simulink model "robust_tracking_integral_REALTIME"  (R2020b)
settings: Solver=ode3  StartTime=0.0  StopTime=5  FixedStep=0.001  RelTol=1e-3
values from neighbouring files (symbols this model uses):
  ctrl =     [PID_params_LAB0.mat]
undefined symbols (not defined in the file or in its folder): degs2rpm, denH1, DiscIntNeverNeededParam, Ke, Ki, N_u, N_x, National_Instruments, numH1, PCI, rpm2rads, sens, step_size
libraries: sldrtlib x3, simulink x2
settings Model: ExtModeTrigDuration=10000  Creator=39345  LastModifiedBy=tortoranic
settings DataIOCC: ReturnWorkspaceOutputs=off
settings RTWCC: Description=Simulink Desktop Real-Time  SystemTargetFile=sldrt.tlc  TemplateMakefile=sldrt.tmf  RTWCompilerOptimization=on
settings CodeAppCC: MaxIdLength=95
settings SimulinkDesktopRealTimeCC: TargetPreCompLibLocation=C:\Program Files\MATLAB\R2020b\toolbox\sldrt\lib\win64

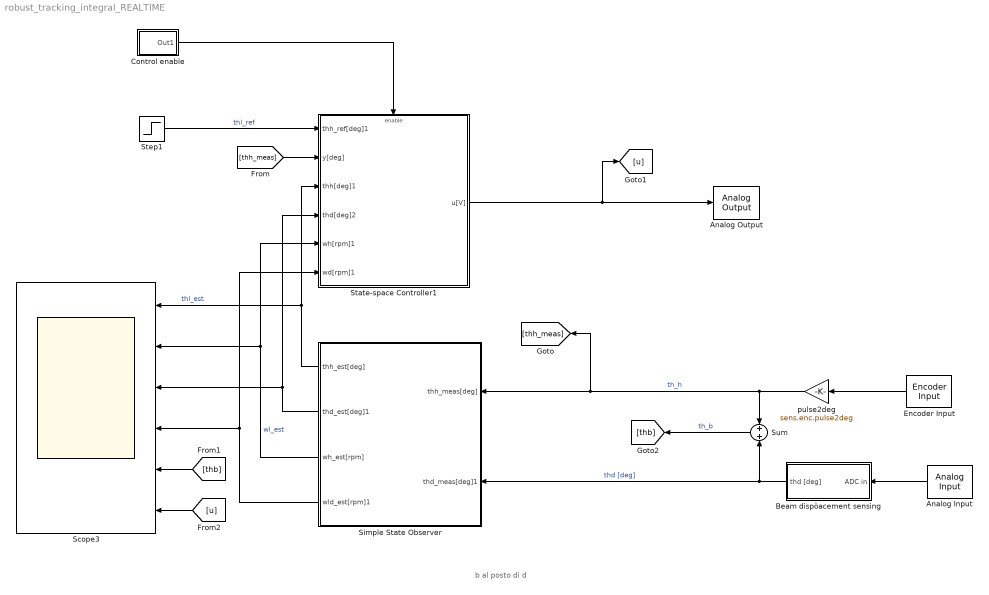
== system robust_tracking_integral_REALTIME ==
  note: b al posto di d
  Analog Input : sldrtlib/Analog Input  SampleTime=0.001  MaxMissedTicks=10  ShowMissedTicks=off  YieldWhenWaiting=off  DrvName=National_Instruments/PCI-6221  DrvAddress=4294967295  DrvOptions=[0 0 0 2 0]  Channels=[3 4]  RangeMode=1  VoltRange=2  DataType=1
      settings: AttributesFormatString=National Instruments\nPCI-6221 [auto]
  Analog Output : sldrtlib/Analog Output  SampleTime=0.001  MaxMissedTicks=10  ShowMissedTicks=off  YieldWhenWaiting=off  DrvName=National_Instruments/PCI-6221  DrvAddress=4294967295  DrvOptions=[0 0 0 2 0]  Channels=1  RangeMode=1  VoltRange=1  InitialValue=0  FinalValue=0
      settings: AttributesFormatString=National Instruments\nPCI-6221 [auto]
  Beam dispòacement sensing : Subsystem
  Control enable : Subsystem
  Encoder Input : sldrtlib/Encoder Input  SampleTime=0.001  MaxMissedTicks=10  ShowMissedTicks=off  YieldWhenWaiting=off  DrvName=National_Instruments/PCI-6221  DrvAddress=4294967295  DrvOptions=[0 0 0 2 0]  Channels=1  QuadMode=3  IndexPulse=1  InputFilter=Inf  DataType=1
      settings: AttributesFormatString=National Instruments\nPCI-6221 [auto]
  Scope3 : Scope  NumInputPorts=6
  Simple State Observer : Subsystem
  State-space Controller1 : Subsystem
  Step1 : Step  After=step_size  SampleTime=0.001
  Sum : Sum
  pulse2deg : Gain  Gain=sens.enc.pulse2deg
  wires:
  Simple State Observer/4(wld_est[rpm]1) -> Scope3/4, State-space Controller1/6(wd[rpm]1)
  Simple State Observer/1(thh_est[deg]) -> Scope3/1, State-space Controller1/3(thh[deg]1)  "thl_est"
  Simple State Observer/3(wh_est[rpm]) -> State-space Controller1/5(wh[rpm]1), Scope3/2  "wl_est"
  Simple State Observer/2(thd_est[deg]1) -> Scope3/3, State-space Controller1/4(thd[deg]2)
  Encoder Input/1 -> pulse2deg/1
  Sum/1 -> [thb]  "th_b"
  [thh_meas] -> State-space Controller1/2(y[deg])
  Step1/1 -> State-space Controller1/1(thh_ref[deg]1)  "thl_ref"
  State-space Controller1/1(u[V]) -> [u], Analog Output/1
  pulse2deg/1 -> Sum/1, [thh_meas], Simple State Observer/1(thh_meas[deg])  "th_h"
  Analog Input/1 -> Beam dispòacement sensing/1(ADC in)
  Beam dispòacement sensing/1(thd [deg]) -> Simple State Observer/2(thd_meas[deg]1), Sum/2  "thd [deg]"
  [thb] -> Scope3/5
  [u] -> Scope3/6
  Control enable/1(Out1) -> State-space Controller1/Enable

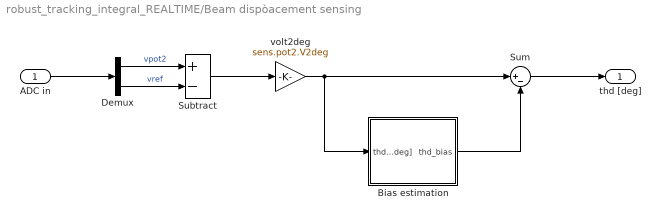
== system robust_tracking_integral_REALTIME/Beam dispòacement sensing ==
  ADC in : Inport
  Bias estimation : Subsystem
  Demux : Demux  Outputs=2
  Subtract : Sum  Inputs=+-
  Sum : Sum  Inputs=|+-
  volt2deg : Gain  Gain=sens.pot2.V2deg
  thd [deg] : Outport
  wires:
  Subtract/1 -> volt2deg/1
  Demux/1 -> Subtract/1  "vpot2"
  Demux/2 -> Subtract/2  "vref"
  ADC in/1 -> Demux/1
  volt2deg/1 -> Bias estimation/1(thd [deg]), Sum/1
  Bias estimation/1(thd_bias) -> Sum/2
  Sum/1 -> thd [deg]/1

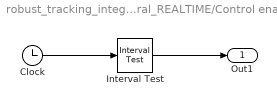
== system robust_tracking_integral_REALTIME/Control enable ==
  Clock : Clock
  Interval Test : simulink/Logic and Bit Operations/Interval Test  IntervalClosedRight=on  uplimit=60  IntervalClosedLeft=on  lowlimit=0.7  OutDataTypeStr=boolean
  Out1 : Outport
  wires:
  Clock/1 -> Interval Test/1
  Interval Test/1 -> Out1/1

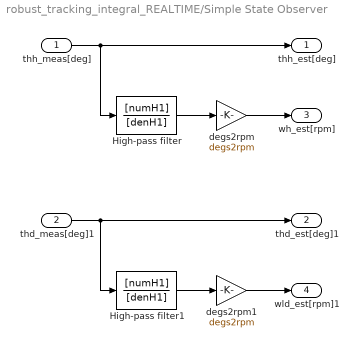
== system robust_tracking_integral_REALTIME/Simple State Observer ==
  thh_meas[deg] : Inport
  thd_meas[deg]1 : Inport  Port=2
  High-pass filter : TransferFcn  Numerator=[numH1]  Denominator=[denH1]
  High-pass filter1 : TransferFcn  Numerator=[numH1]  Denominator=[denH1]
  degs2rpm : Gain  Gain=degs2rpm
  degs2rpm1 : Gain  Gain=degs2rpm
  thh_est[deg] : Outport
  thd_est[deg]1 : Outport  Port=2
  wh_est[rpm] : Outport  Port=3
  wld_est[rpm]1 : Outport  Port=4
  wires:
  thh_meas[deg]/1 -> thh_est[deg]/1, High-pass filter/1
  High-pass filter/1 -> degs2rpm/1
  degs2rpm/1 -> wh_est[rpm]/1
  thd_meas[deg]1/1 -> thd_est[deg]1/1, High-pass filter1/1
  High-pass filter1/1 -> degs2rpm1/1
  degs2rpm1/1 -> wld_est[rpm]1/1

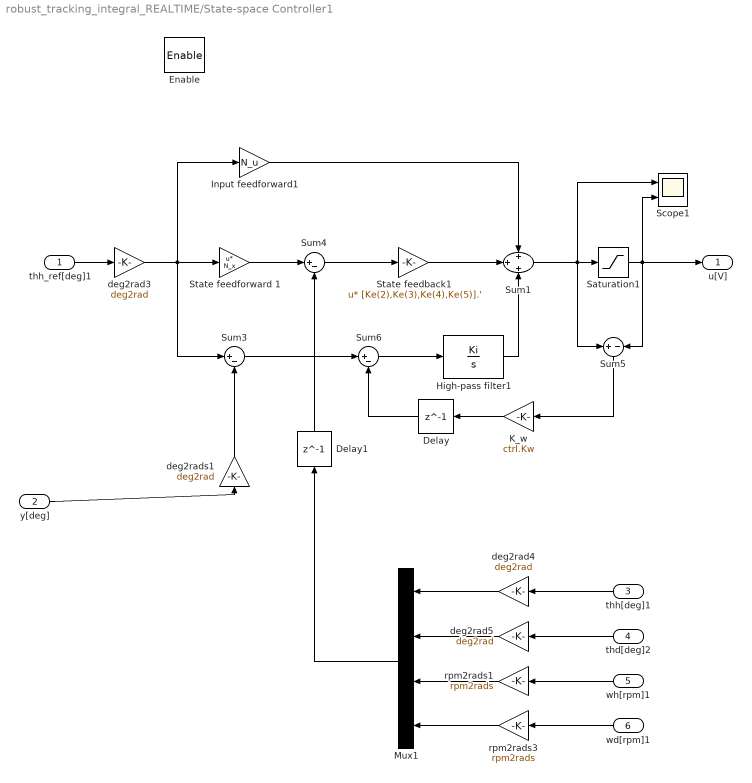
== system robust_tracking_integral_REALTIME/State-space Controller1 ==
  thh_ref[deg]1 : Inport
  y[deg] : Inport  Port=2
  thh[deg]1 : Inport  Port=3
  thd[deg]2 : Inport  Port=4
  wh[rpm]1 : Inport  Port=5
  wd[rpm]1 : Inport  Port=6
  Enable : EnablePort
  Delay : Delay  DelayLength=1  InitialCondition=0
  Delay1 : Delay  DelayLength=1  InitialCondition=0
  High-pass filter1 : TransferFcn  Numerator=Ki  Denominator=[1 0]
  Input feedforward1 : Gain  Gain=N_u
  K_w : Gain  Gain=ctrl.Kw
  Mux1 : Mux
  Saturation1 : Saturate  UpperLimit=10  LowerLimit=-10
  Scope1 : Scope  NumInputPorts=2
  State feedback1 : Gain  Gain=[Ke(2),Ke(3),Ke(4),Ke(5)].'  Multiplication=Matrix(u*K)
  State feedforward	1 : Gain  Gain=N_x  Multiplication=Matrix(u*K)
  Sum1 : Sum  Inputs=+|+|+
  Sum3 : Sum  Inputs=|+-
  Sum4 : Sum  Inputs=|+-
  Sum5 : Sum  Inputs=+|-
  Sum6 : Sum  Inputs=|+-
  deg2rad3 : Gain  Gain=deg2rad
  deg2rad4 : Gain  Gain=deg2rad
  deg2rad5 : Gain  Gain=deg2rad
  deg2rads1 : Gain  Gain=deg2rad
  rpm2rads1 : Gain  Gain=rpm2rads
  rpm2rads3 : Gain  Gain=rpm2rads
  u[V] : Outport
  wires:
  Delay/1 -> Sum6/2
  Sum6/1 -> High-pass filter1/1
  deg2rads1/1 -> Sum3/2
  y[deg]/1 -> deg2rads1/1
  Sum1/1 -> Sum5/1, Scope1/1, Saturation1/1
  Delay1/1 -> Sum4/2
  K_w/1 -> Delay/1
  High-pass filter1/1 -> Sum1/3
  Sum5/1 -> K_w/1
  Sum3/1 -> Sum6/1
  State feedback1/1 -> Sum1/2
  Sum4/1 -> State feedback1/1
  deg2rad3/1 -> Sum3/1, Input feedforward1/1, State feedforward	1/1
  Saturation1/1 -> Sum5/2, Scope1/2, u[V]/1
  State feedforward	1/1 -> Sum4/1
  Input feedforward1/1 -> Sum1/1
  deg2rad5/1 -> Mux1/2
  Mux1/1 -> Delay1/1
  rpm2rads1/1 -> Mux1/3
  wd[rpm]1/1 -> rpm2rads3/1
  wh[rpm]1/1 -> rpm2rads1/1
  thh[deg]1/1 -> deg2rad4/1
  deg2rad4/1 -> Mux1/1
  thd[deg]2/1 -> deg2rad5/1
  rpm2rads3/1 -> Mux1/4
  thh_ref[deg]1/1 -> deg2rad3/1

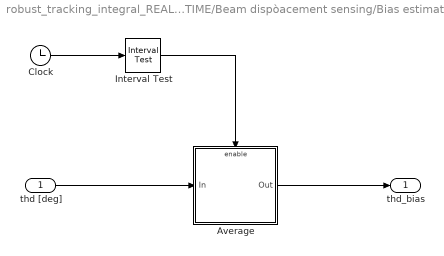
== system robust_tracking_integral_REALTIME/Beam dispòacement sensing/Bias estimation ==
  thd [deg] : Inport
  Average : Subsystem
  Clock : Clock
  Interval Test : simulink/Logic and Bit Operations/Interval Test  IntervalClosedRight=on  uplimit=0.7  IntervalClosedLeft=on  lowlimit=0.2  OutDataTypeStr=boolean
  thd_bias : Outport
  wires:
  Clock/1 -> Interval Test/1
  thd [deg]/1 -> Average/1(In)
  Average/1(Out) -> thd_bias/1
  Interval Test/1 -> Average/Enable

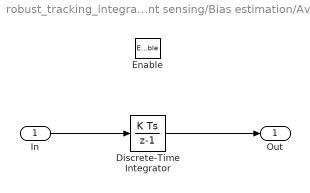
== system robust_tracking_integral_REALTIME/Beam dispòacement sensing/Bias estimation/Average ==
  In : Inport
  Enable : EnablePort
  Discrete-Time Integrator : DiscreteIntegrator  gainval=2.0  SampleTime=0.001  ICPrevOutput=DiscIntNeverNeededParam  ICPrevScaledInput=DiscIntNeverNeededParam
  Out : Outport
  wires:
  In/1 -> Discrete-Time Integrator/1
  Discrete-Time Integrator/1 -> Out/1
